simulink model "task2a"  (R2018b)
settings: Solver=VariableStepAuto  StartTime=0.0  StopTime=10.0  RelTol=1e-3
settings Model: Creator=root  LastModifiedBy=root

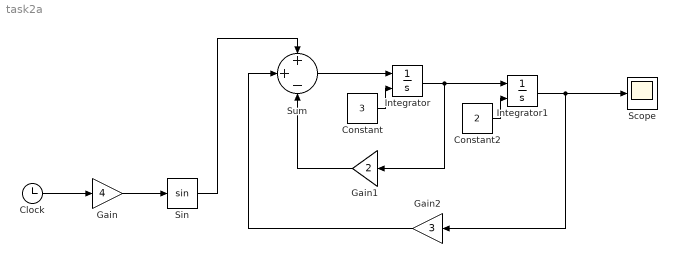
== system task2a ==
  Clock : Clock
  Constant : Constant  Value=3
  Constant2 : Constant  Value=2
  Gain : Gain  Gain=4
  Gain1 : Gain  Gain=2
  Gain2 : Gain  Gain=3
  Integrator : Integrator  InitialConditionSource=external  InitialCondition=1
  Integrator1 : Integrator  InitialConditionSource=external  InitialCondition=1
  Scope : Scope
  Sin : Trigonometry
  Sum : Sum  Inputs=++-
  wires:
  Clock/1 -> Gain/1
  Gain/1 -> Sin/1
  Sin/1 -> Sum/1
  Constant/1 -> Integrator/2
  Sum/1 -> Integrator/1
  Constant2/1 -> Integrator1/2
  Integrator/1 -> Gain1/1, Integrator1/1
  Gain1/1 -> Sum/3
  Integrator1/1 -> Gain2/1, Scope/1
  Gain2/1 -> Sum/2
